simulink model "IEEE123bus_v2019b_Phasor_PI"  (R2019b)
settings: Solver=ode4  StartTime=0.0  StopTime=100  FixedStep=Ts  MaxStep=1e-4  RelTol=1e-3
InitFcn:
  | a=1; % Loading Factor
  | Ts=0.1;% For Delay Blocks in Voltage Regulator Controls
  | % phase to sequence conversion of RXB matrices
  | c=1*exp(sqrt(-1)*(120*pi/180));
  | T=[1 1 1;1 c*c c;1 c c*c];
  | Tinv=1/3*[1 1 1;1 c c*c;1 c*c c];
  | 
  | % Simulation data for the IEEE 123 Node Test Feeder model
  | mi2km = 1.60934;%  miles to km conversion
  | ft2km = 0.0003048; % feet to km conversion
  | ms2F = 1*1e-6/(2*pi*60);% microsiemens to Farads conversion
  | 
  | %% Configuration 1
  | % Series Resitance and Reactance - ohm/mile
  | R_1 = [0.4576 0.1560 0.1535;0.1560 0.4666 0.1580;0.1535 0.1580 0.4615];
  | X_1 = [1.0780 0.5017 0.3849;0.5017 1.0482 0.4236;0.3849 0.4236 1.0651];
  | % charging susceptance - microsiemens/mile
  | B_1 = [5.6765 -1.8319 -0.6982;-1.8319 5.9809 -1.1645;-0.6982 -1.1645 5.3971];
  | 
  | R_1 = R_1/mi2km;
  | Rseq=Tinv*R_1*T;
  | R1_1=Rseq(2,2);R0_1=Rseq(1,1);
  | 
  | L_1 = (X_1/(2*pi*60))/mi2km;
  | Lseq=Tinv*L_1*T;
  | L1_1=Lseq(2,2);L0_1=Lseq(1,1);
  | 
  | C_1 =(B_1*ms2F)/mi2km;
  | Cseq=Tinv*C_1*T;
  | C1_1=Cseq(2,2);C0_1=Cseq(1,1);
  | %% Configuration 2 - series reactance - ohm/mile
  | R_2 = [0.4666 0.1580 0.1560;0.1580 0.4615 0.1535;0.1560 0.1535 0.4576];
  | X_2 = [1.0482 0.4236 0.5017;0.4236 1.0651 0.3849;0.5017 0.3849 1.0780];
  | % charging susceptance - microsiemens/mile
  | B_2 = [5.9809 -1.1645 -1.8319;-1.1645 5.3971 -0.6982;-1.8319 -0.6982 5.6765];
  | 
  | R_2 = R_2/mi2km;
  | Rseq=Tinv*R_2*T;
  | R1_2=Rseq(2,2);R0_2=Rseq(1,1);
  | 
  | L_2 = (X_2/(2*pi*60))/mi2km;
  | Lseq=Tinv*L_2*T;
  | L1_2=Lseq(2,2);L0_2=Lseq(1,1);
  | 
  | C_2 =(B_2*ms2F)/mi2km;
  | Cseq=Tinv*C_2*T;
  | C1_2=Cseq(2,2);C0_2=Cseq(1,1);
  | %% Configuration 3 - series reactance - ohm/mile
  | R_3 = [0.4615 0.1535 0.1580;0.1535 0.4576 0.1560;0.1580 0.1560 0.4666];
  | X_3 = [1.0651 0.3849 0.4236;0.3849 1.0780 0.5017;0.4236 0.5017 1.0482];
  | % charging susceptance - microsiemens/mile
  | B_3 = [5.3971 -0.6982 -1.1645;-0.6982 5.6765 -1.8319; -1.1645 -1.8319 5.9809];
  | 
  | R_3 = R_3/mi2km;
  | Rseq=Tinv*R_3*T;
  | R1_3=Rseq(2,2);R0_3=Rseq(1,1);
  | 
  | L_3 = (X_3/(2*pi*60))/mi2km;
  | Lseq=Tinv*L_3*T;
  | L1_3=Lseq(2,2);L0_3=Lseq(1,1);
  | ... (+157 lines)
undefined symbols (not defined in the file or in its folder): D1, Delta, find_system, j
libraries: powerlib x771, powerlib_meascontrol x31
(part 4 of 7)

== system IEEE123bus_v2019b_Phasor_PI/Regulator 3 ==
  Mux : Mux  Inputs=2
  Single Phase SVR_A : Subsystem  LoadFcn=find_system(gcs,'FollowLinks', 'on', 'LookUnderMasks', 'all');  mask(Single-Phase OLTC){pNom=5e6/3, fNom=60, vNom=4160/sqrt(3), ctRatio=50, ptRatio=20, DeltaU=0.00625, TapMinMax=[-16 16], InitialTap=0, TapSelectionTime=8, RegulatorOn=on, Regulator=[120/120  1/120  12], Comp=[0.4 0.4]}
      mask prompts: pNom "Nominal Power (VA)"; fNom "Nominal Frequency (Hz)"; vNom "Nominal Voltage (Vrms)"; ctRatio "Primary CT Rating (A)"; ptRatio "PT Ratio"; DeltaU "Voltage Step Per Tap (pu)"; TapMinMax "Minimum and Maximum Tap Positions"; InitialTap "Initial Tap Position"; TapSelectionTime "Tap Selection Time (s)"; RegulatorOn "Voltage Regulator"; Regulator "Voltage Regulator [ Vref(pu) DeadBand(pu)  Delay(s)]"; Comp "Compensator Settings [R (V) X(V)]"
      mask help:
      | Models a single-phase On Load Tap Changer (OLTC). The single-phase primary of multi-tap winding is modeled with a Variable-Ratio Transformer block.
      |
      | The transformer voltage ratio U2/U1 (in pu) is given by:
      |                 U2/U1= 1/ (1+TapPosition*DeltaU)
      | Tap position 0 corresponds to nominal voltage ratio.
      |
      | When Voltage regulator is 'on',  voltage regulator asks for a tap change if:
      |                  abs(Vm-Vref)>DeadBand/2  during a time  t > Delay.
      |
      | where 'Vm' is voltage measured at regulating point and Vref is reference voltage.
      | With line drop compensation, Vm=Vsec-Isec(R+jX)
      mask init:
      | RegulatorVref=Regulator(1);
      | RegulatorDeadBand=Regulator(2);
      | RegulatorDelay=Regulator(3);
      | Rc=Comp(1);
      | Xc=Comp(2);
      mask TypeOptions RegulatorOn: off | on
      mask Callback RegulatorOn:
      | tempMaskVis=get_param(gcb,'MaskVisibilities');
      | if strcmp(get_param(gcb,'RegulatorOn'),'on')
      | 	tempMaskVis{11}='on';
      | 	set_param(gcb,'MaskVisibilities',tempMaskVis);
      | else
      | 	tempMaskVis{11}='off';
      | 	set_param(gcb,'MaskVisibilities',tempMaskVis);
      | end
      | if strcmp(get_param(gcb,'RegulatorOn'),'on')
      | 	tempMaskVis{12}='on';
      | 	set_param(gcb,'MaskVisibilities',tempMaskVis);
      | else
      | 	tempMaskVis{12}='off';
      | 	set_param(gcb,'MaskVisibilities',tempMaskVis);
      | end
      mask DialogControl Container8 Prompt: Setup
      mask DialogControl Container13 Prompt: Regulator Parameters
  Single Phase SVR_C : Subsystem  LoadFcn=find_system(gcs,'FollowLinks', 'on', 'LookUnderMasks', 'all');  mask(Single-Phase OLTC){pNom=5e6/3, fNom=60, vNom=4160/sqrt(3), ctRatio=50, ptRatio=20, DeltaU=0.00625, TapMinMax=[-16 16], InitialTap=-1, TapSelectionTime=8, RegulatorOn=on, Regulator=[120/120  1/120  12], Comp=[0.4 0.4]}
      mask prompts: pNom "Nominal Power (VA)"; fNom "Nominal Frequency (Hz)"; vNom "Nominal Voltage (Vrms)"; ctRatio "Primary CT Rating (A)"; ptRatio "PT Ratio"; DeltaU "Voltage Step Per Tap (pu)"; TapMinMax "Minimum and Maximum Tap Positions"; InitialTap "Initial Tap Position"; TapSelectionTime "Tap Selection Time (s)"; RegulatorOn "Voltage Regulator"; Regulator "Voltage Regulator [ Vref(pu) DeadBand(pu)  Delay(s)]"; Comp "Compensator Settings [R (V) X(V)]"
      mask help:
      | Models a single-phase On Load Tap Changer (OLTC). The single-phase primary of multi-tap winding is modeled with a Variable-Ratio Transformer block.
      |
      | The transformer voltage ratio U2/U1 (in pu) is given by:
      |                 U2/U1= 1/ (1+TapPosition*DeltaU)
      | Tap position 0 corresponds to nominal voltage ratio.
      |
      | When Voltage regulator is 'on',  voltage regulator asks for a tap change if:
      |                  abs(Vm-Vref)>DeadBand/2  during a time  t > Delay.
      |
      | where 'Vm' is voltage measured at regulating point and Vref is reference voltage.
      | With line drop compensation, Vm=Vsec-Isec(R+jX)
      mask init:
      | RegulatorVref=Regulator(1);
      | RegulatorDeadBand=Regulator(2);
      | RegulatorDelay=Regulator(3);
      | Rc=Comp(1);
      | Xc=Comp(2);
      mask TypeOptions RegulatorOn: off | on
      mask Callback RegulatorOn:
      | tempMaskVis=get_param(gcb,'MaskVisibilities');
      | if strcmp(get_param(gcb,'RegulatorOn'),'on')
      | 	tempMaskVis{11}='on';
      | 	set_param(gcb,'MaskVisibilities',tempMaskVis);
      | else
      | 	tempMaskVis{11}='off';
      | 	set_param(gcb,'MaskVisibilities',tempMaskVis);
      | end
      | if strcmp(get_param(gcb,'RegulatorOn'),'on')
      | 	tempMaskVis{12}='on';
      | 	set_param(gcb,'MaskVisibilities',tempMaskVis);
      | else
      | 	tempMaskVis{12}='off';
      | 	set_param(gcb,'MaskVisibilities',tempMaskVis);
      | end
      mask DialogControl Container8 Prompt: Setup
      mask DialogControl Container13 Prompt: Regulator Parameters
  A : PMIOPort  Side=Left
  a : PMIOPort  Port=2  Side=Right
  C : PMIOPort  Port=3  Side=Left
  c : PMIOPort  Port=4  Side=Right
  Taps : Outport
  wires:
  Single Phase SVR_A/1(Tap) -> Mux/1
  Single Phase SVR_C/1(Tap) -> Mux/2
  Mux/1 -> Taps/1
  connections:
  Single Phase SVR_A/LConn1 -- A/RConn1
  Single Phase SVR_C/LConn1 -- C/RConn1
  Single Phase SVR_A/RConn1 -- a/RConn1
  Single Phase SVR_C/RConn1 -- c/RConn1

== system IEEE123bus_v2019b_Phasor_PI/Regulator 4 ==
  Mux : Mux  Inputs=3
  Single Phase SVR_A : Subsystem  LoadFcn=find_system(gcs,'FollowLinks', 'on', 'LookUnderMasks', 'all');  mask(Single-Phase OLTC){pNom=5e6/3, fNom=60, vNom=4160/sqrt(3), ctRatio=300, ptRatio=20, DeltaU=0.00625, TapMinMax=[-16 16], InitialTap=8, TapSelectionTime=8, RegulatorOn=on, Regulator=[124/120  2/120  12], Comp=[0.6 1.3]}
      mask prompts: pNom "Nominal Power (VA)"; fNom "Nominal Frequency (Hz)"; vNom "Nominal Voltage (Vrms)"; ctRatio "Primary CT Rating (A)"; ptRatio "PT Ratio"; DeltaU "Voltage Step Per Tap (pu)"; TapMinMax "Minimum and Maximum Tap Positions"; InitialTap "Initial Tap Position"; TapSelectionTime "Tap Selection Time (s)"; RegulatorOn "Voltage Regulator"; Regulator "Voltage Regulator [ Vref(pu) DeadBand(pu)  Delay(s)]"; Comp "Compensator Settings [R (V) X(V)]"
      mask help:
      | Models a single-phase On Load Tap Changer (OLTC). The single-phase primary of multi-tap winding is modeled with a Variable-Ratio Transformer block.
      |
      | The transformer voltage ratio U2/U1 (in pu) is given by:
      |                 U2/U1= 1/ (1+TapPosition*DeltaU)
      | Tap position 0 corresponds to nominal voltage ratio.
      |
      | When Voltage regulator is 'on',  voltage regulator asks for a tap change if:
      |                  abs(Vm-Vref)>DeadBand/2  during a time  t > Delay.
      |
      | where 'Vm' is voltage measured at regulating point and Vref is reference voltage.
      | With line drop compensation, Vm=Vsec-Isec(R+jX)
      mask init:
      | RegulatorVref=Regulator(1);
      | RegulatorDeadBand=Regulator(2);
      | RegulatorDelay=Regulator(3);
      | Rc=Comp(1);
      | Xc=Comp(2);
      mask TypeOptions RegulatorOn: off | on
      mask Callback RegulatorOn:
      | tempMaskVis=get_param(gcb,'MaskVisibilities');
      | if strcmp(get_param(gcb,'RegulatorOn'),'on')
      | 	tempMaskVis{11}='on';
      | 	set_param(gcb,'MaskVisibilities',tempMaskVis);
      | else
      | 	tempMaskVis{11}='off';
      | 	set_param(gcb,'MaskVisibilities',tempMaskVis);
      | end
      | if strcmp(get_param(gcb,'RegulatorOn'),'on')
      | 	tempMaskVis{12}='on';
      | 	set_param(gcb,'MaskVisibilities',tempMaskVis);
      | else
      | 	tempMaskVis{12}='off';
      | 	set_param(gcb,'MaskVisibilities',tempMaskVis);
      | end
      mask DialogControl Container8 Prompt: Setup
      mask DialogControl Container13 Prompt: Regulator Parameters
  Single Phase SVR_B : Subsystem  LoadFcn=find_system(gcs,'FollowLinks', 'on', 'LookUnderMasks', 'all');  mask(Single-Phase OLTC){pNom=5e6/3, fNom=60, vNom=4160/sqrt(3), ctRatio=300, ptRatio=20, DeltaU=0.00625, TapMinMax=[-16 16], InitialTap=1, TapSelectionTime=8, RegulatorOn=on, Regulator=[124/120  2/120  12], Comp=[0.6 1.3]}
      mask prompts: pNom "Nominal Power (VA)"; fNom "Nominal Frequency (Hz)"; vNom "Nominal Voltage (Vrms)"; ctRatio "Primary CT Rating (A)"; ptRatio "PT Ratio"; DeltaU "Voltage Step Per Tap (pu)"; TapMinMax "Minimum and Maximum Tap Positions"; InitialTap "Initial Tap Position"; TapSelectionTime "Tap Selection Time (s)"; RegulatorOn "Voltage Regulator"; Regulator "Voltage Regulator [ Vref(pu) DeadBand(pu)  Delay(s)]"; Comp "Compensator Settings [R (V) X(V)]"
      mask help:
      | Models a single-phase On Load Tap Changer (OLTC). The single-phase primary of multi-tap winding is modeled with a Variable-Ratio Transformer block.
      |
      | The transformer voltage ratio U2/U1 (in pu) is given by:
      |                 U2/U1= 1/ (1+TapPosition*DeltaU)
      | Tap position 0 corresponds to nominal voltage ratio.
      |
      | When Voltage regulator is 'on',  voltage regulator asks for a tap change if:
      |                  abs(Vm-Vref)>DeadBand/2  during a time  t > Delay.
      |
      | where 'Vm' is voltage measured at regulating point and Vref is reference voltage.
      | With line drop compensation, Vm=Vsec-Isec(R+jX)
      mask init:
      | RegulatorVref=Regulator(1);
      | RegulatorDeadBand=Regulator(2);
      | RegulatorDelay=Regulator(3);
      | Rc=Comp(1);
      | Xc=Comp(2);
      mask TypeOptions RegulatorOn: off | on
      mask Callback RegulatorOn:
      | tempMaskVis=get_param(gcb,'MaskVisibilities');
      | if strcmp(get_param(gcb,'RegulatorOn'),'on')
      | 	tempMaskVis{11}='on';
      | 	set_param(gcb,'MaskVisibilities',tempMaskVis);
      | else
      | 	tempMaskVis{11}='off';
      | 	set_param(gcb,'MaskVisibilities',tempMaskVis);
      | end
      | if strcmp(get_param(gcb,'RegulatorOn'),'on')
      | 	tempMaskVis{12}='on';
      | 	set_param(gcb,'MaskVisibilities',tempMaskVis);
      | else
      | 	tempMaskVis{12}='off';
      | 	set_param(gcb,'MaskVisibilities',tempMaskVis);
      | end
      mask DialogControl Container8 Prompt: Setup
      mask DialogControl Container13 Prompt: Regulator Parameters
  Single Phase SVR_C : Subsystem  LoadFcn=find_system(gcs,'FollowLinks', 'on', 'LookUnderMasks', 'all');  mask(Single-Phase OLTC){pNom=5e6/3, fNom=60, vNom=4160/sqrt(3), ctRatio=300, ptRatio=20, DeltaU=0.00625, TapMinMax=[-16 16], InitialTap=5, TapSelectionTime=8, RegulatorOn=on, Regulator=[124/120  2/120  12], Comp=[0.6 1.3]}
      mask prompts: pNom "Nominal Power (VA)"; fNom "Nominal Frequency (Hz)"; vNom "Nominal Voltage (Vrms)"; ctRatio "Primary CT Rating (A)"; ptRatio "PT Ratio"; DeltaU "Voltage Step Per Tap (pu)"; TapMinMax "Minimum and Maximum Tap Positions"; InitialTap "Initial Tap Position"; TapSelectionTime "Tap Selection Time (s)"; RegulatorOn "Voltage Regulator"; Regulator "Voltage Regulator [ Vref(pu) DeadBand(pu)  Delay(s)]"; Comp "Compensator Settings [R (V) X(V)]"
      mask help:
      | Models a single-phase On Load Tap Changer (OLTC). The single-phase primary of multi-tap winding is modeled with a Variable-Ratio Transformer block.
      |
      | The transformer voltage ratio U2/U1 (in pu) is given by:
      |                 U2/U1= 1/ (1+TapPosition*DeltaU)
      | Tap position 0 corresponds to nominal voltage ratio.
      |
      | When Voltage regulator is 'on',  voltage regulator asks for a tap change if:
      |                  abs(Vm-Vref)>DeadBand/2  during a time  t > Delay.
      |
      | where 'Vm' is voltage measured at regulating point and Vref is reference voltage.
      | With line drop compensation, Vm=Vsec-Isec(R+jX)
      mask init:
      | RegulatorVref=Regulator(1);
      | RegulatorDeadBand=Regulator(2);
      | RegulatorDelay=Regulator(3);
      | Rc=Comp(1);
      | Xc=Comp(2);
      mask TypeOptions RegulatorOn: off | on
      mask Callback RegulatorOn:
      | tempMaskVis=get_param(gcb,'MaskVisibilities');
      | if strcmp(get_param(gcb,'RegulatorOn'),'on')
      | 	tempMaskVis{11}='on';
      | 	set_param(gcb,'MaskVisibilities',tempMaskVis);
      | else
      | 	tempMaskVis{11}='off';
      | 	set_param(gcb,'MaskVisibilities',tempMaskVis);
      | end
      | if strcmp(get_param(gcb,'RegulatorOn'),'on')
      | 	tempMaskVis{12}='on';
      | 	set_param(gcb,'MaskVisibilities',tempMaskVis);
      | else
      | 	tempMaskVis{12}='off';
      | 	set_param(gcb,'MaskVisibilities',tempMaskVis);
      | end
      mask DialogControl Container8 Prompt: Setup
      mask DialogControl Container13 Prompt: Regulator Parameters
  A : PMIOPort  Side=Left
  a : PMIOPort  Port=2  Side=Right
  B : PMIOPort  Port=3  Side=Left
  b : PMIOPort  Port=4  Side=Right
  C : PMIOPort  Port=5  Side=Left
  c : PMIOPort  Port=6  Side=Right
  Tap : Outport
  wires:
  Mux/1 -> Tap/1
  Single Phase SVR_C/1(Tap) -> Mux/3
  Single Phase SVR_B/1(Tap) -> Mux/2
  Single Phase SVR_A/1(Tap) -> Mux/1
  connections:
  Single Phase SVR_C/RConn1 -- c/RConn1
  Single Phase SVR_C/LConn1 -- C/RConn1
  Single Phase SVR_B/RConn1 -- b/RConn1
  Single Phase SVR_B/LConn1 -- B/RConn1
  Single Phase SVR_A/LConn1 -- A/RConn1
  Single Phase SVR_A/RConn1 -- a/RConn1

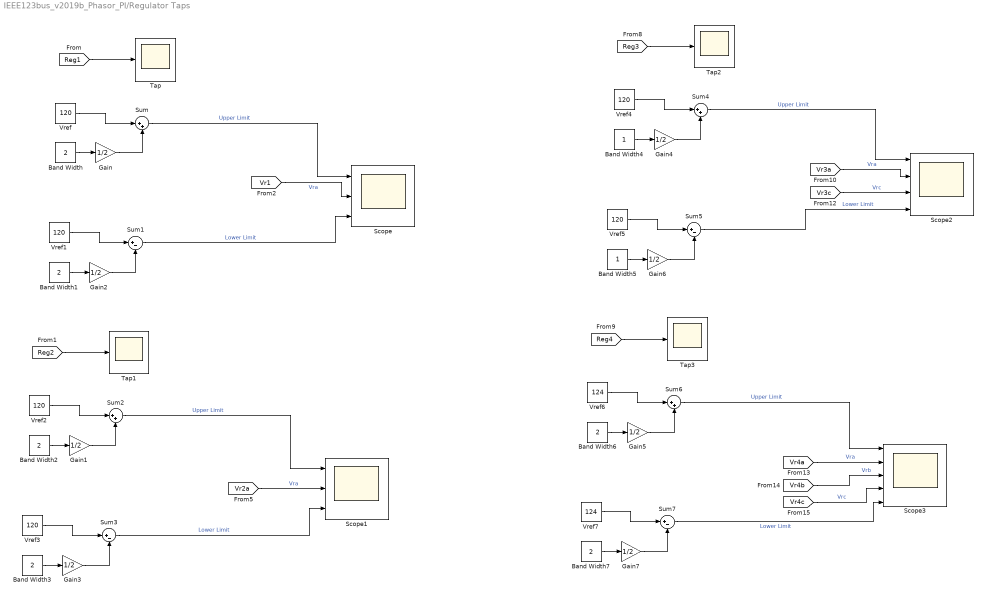
== system IEEE123bus_v2019b_Phasor_PI/Regulator Taps ==
  Band Width{,1..3,6..7} (6 alike) : Constant  Value=2
  Band Width4 : Constant
  Band Width5 : Constant
  Gain{,1..7} (8 alike) : Gain  Gain=1/2
  Scope : Scope  NumInputPorts=3
  Scope1 : Scope  NumInputPorts=3
  Scope2 : Scope  NumInputPorts=4
  Scope3 : Scope  NumInputPorts=5
  Sum{,2,4,6} (4 alike) : Sum  Inputs=|++
  Sum{1,3,5,7} (4 alike) : Sum  Inputs=|+-
  Tap{,1..3} (4 alike) : Scope
  Vref{,1..5} (6 alike) : Constant  Value=120
  Vref6 : Constant  Value=124
  Vref7 : Constant  Value=124
  wires:
  Vref/1 -> Sum/1
  Gain2/1 -> Sum1/2
  Band Width/1 -> Gain/1
  Gain/1 -> Sum/2
  [Reg1] -> Tap/1
  Band Width1/1 -> Gain2/1
  Sum/1 -> Scope/1  "Upper Limit"
  Vref1/1 -> Sum1/1
  Sum1/1 -> Scope/3  "Lower Limit"
  [Vr1] -> Scope/2  "Vra"
  [Vr2a] -> Scope1/2  "Vra"
  Sum3/1 -> Scope1/3  "Lower Limit"
  Vref3/1 -> Sum3/1
  Sum2/1 -> Scope1/1  "Upper Limit"
  Band Width3/1 -> Gain3/1
  [Reg2] -> Tap1/1
  Gain1/1 -> Sum2/2
  Band Width2/1 -> Gain1/1
  Gain3/1 -> Sum3/2
  Vref2/1 -> Sum2/1
  Vref6/1 -> Sum6/1
  Gain7/1 -> Sum7/2
  Band Width6/1 -> Gain5/1
  Gain5/1 -> Sum6/2
  [Reg4] -> Tap3/1
  [Vr4c] -> Scope3/4  "Vrc"
  Band Width7/1 -> Gain7/1
  Sum6/1 -> Scope3/1  "Upper Limit"
  Vref7/1 -> Sum7/1
  Sum7/1 -> Scope3/5  "Lower Limit"
  [Vr4b] -> Scope3/3  "Vrb"
  [Vr4a] -> Scope3/2  "Vra"
  [Vr3a] -> Scope2/2  "Vra"
  Sum5/1 -> Scope2/4  "Lower Limit"
  Vref5/1 -> Sum5/1
  Sum4/1 -> Scope2/1  "Upper Limit"
  Band Width5/1 -> Gain6/1
  [Vr3c] -> Scope2/3  "Vrc"
  [Reg3] -> Tap2/1
  Gain4/1 -> Sum4/2
  Band Width4/1 -> Gain4/1
  Gain6/1 -> Sum5/2
  Vref4/1 -> Sum4/1

== system IEEE123bus_v2019b_Phasor_PI/Substation Power ==
  note: TOTAL
  note: From Benchmark Document
      |
      | SYSTEM PHASE PHASE PHASE TOTAL
      | INPUT -------(A)-------|-------(B)-------|-------(C)-------|------------------
      | kW : 1463.861 | 963.484 | 1193.153 | 3620.498
      | kVAr : 582.101 | 343.687 | 398.976 | 1324.765
  note: PHASE A
  note: PHASE B
  note: PHASE C
  Demux : Demux  Outputs=3
  Demux1 : Demux  Outputs=3
  Display{,1..7} (8 alike) : Display
  Gain{,1..7} (8 alike) : Gain  Gain=1e-3
  "Power (3ph, Phasor)" : powerlib_meascontrol/Measurements/Power (3ph, Phasor)
      settings: SourceProductName=Simscape Electrical  SourceProductBaseCode=PS
  Power (Phasor) : powerlib_meascontrol/Measurements/Power (Phasor)
      settings: SourceProductName=Simscape Electrical  SourceProductBaseCode=PS
  Power (Phasor)1 : powerlib_meascontrol/Measurements/Power (Phasor)
      settings: SourceProductName=Simscape Electrical  SourceProductBaseCode=PS
  Power (Phasor)2 : powerlib_meascontrol/Measurements/Power (Phasor)
      settings: SourceProductName=Simscape Electrical  SourceProductBaseCode=PS
  wires:
  [I150] -> "Power (3ph, Phasor)"/2
  [V150] -> "Power (3ph, Phasor)"/1
  "Power (3ph, Phasor)"/1 -> Gain/1
  "Power (3ph, Phasor)"/2 -> Gain1/1
  [V150] -> Demux/1
  [I150] -> Demux1/1
  Demux/1 -> Power (Phasor)/1
  Demux1/1 -> Power (Phasor)/2
  Demux/2 -> Power (Phasor)1/1
  Demux1/2 -> Power (Phasor)1/2
  Demux/3 -> Power (Phasor)2/1
  Demux1/3 -> Power (Phasor)2/2
  Power (Phasor)/1 -> Gain2/1
  Power (Phasor)/2 -> Gain3/1
  Power (Phasor)1/1 -> Gain4/1
  Power (Phasor)1/2 -> Gain5/1
  Power (Phasor)2/1 -> Gain6/1
  Power (Phasor)2/2 -> Gain7/1
  Gain/1 -> Display/1
  Gain1/1 -> Display1/1
  Gain2/1 -> Display2/1
  Gain3/1 -> Display3/1
  Gain4/1 -> Display4/1
  Gain5/1 -> Display5/1
  Gain6/1 -> Display6/1
  Gain7/1 -> Display7/1

== system IEEE123bus_v2019b_Phasor_PI/Regulator 1/Single Phase SVR_A ==
  Line Drop Compensator : Subsystem
  Transformer with Taps : Subsystem
  Voltage Regulator Control : Subsystem
  S : PMIOPort  Tag=PMCPort  Side=Left
  L : PMIOPort  Tag=PMCPort  Port=2  Side=Right
  Tap : Outport  VectorParamsAs1DForOutWhenUnconnected=off
  tag scope: Vr2a=global
  wires:
  Line Drop Compensator/1(Vm) -> Voltage Regulator Control/1(Vm), [Vr2a]
  Voltage Regulator Control/1(Tap) -> Transformer with Taps/1(tap), Tap/1
  Transformer with Taps/1(Isec) -> Line Drop Compensator/1(Isec)
  Transformer with Taps/2(Vsec) -> Line Drop Compensator/2(Vsec)
  connections:
  Transformer with Taps/RConn1 -- L/RConn1
  Transformer with Taps/LConn1 -- S/RConn1

== system IEEE123bus_v2019b_Phasor_PI/Regulator 1 Three Phase Ganged SVR/Ganged Line Drop Compensator ==
  note: Vm=Vsec-Isec(Rc+jXc)
  Isec : Inport
  Vsec : Inport  Port=2
  Abs1 : Abs
  Gain4 : Gain  Gain=1/sqrt(2)
  Gain5 : Gain  Gain=Rc+j*Xc
  Gain6 : Gain  Gain=1/sqrt(2)
  Sum1 : Sum  Inputs=|+-
  Vm : Outport
  wires:
  Abs1/1 -> Vm/1
  Gain5/1 -> Sum1/2
  Isec/1 -> Gain4/1
  Gain4/1 -> Gain5/1
  Gain6/1 -> Sum1/1
  Sum1/1 -> Abs1/1
  Vsec/1 -> Gain6/1

== system IEEE123bus_v2019b_Phasor_PI/Regulator 1 Three Phase Ganged SVR/Single Phase SVR_A ==
  Vm : Inport
  Transformer with Taps : Subsystem
  Voltage Regulator Control : Subsystem
  S : PMIOPort  Tag=PMCPort  Side=Left
  L : PMIOPort  Tag=PMCPort  Port=2  Side=Right
  Tap : Outport  VectorParamsAs1DForOutWhenUnconnected=off
  Isec : Outport  Port=2  VectorParamsAs1DForOutWhenUnconnected=off
  Vsec : Outport  Port=3  VectorParamsAs1DForOutWhenUnconnected=off
  wires:
  Transformer with Taps/2(Vsec) -> Vsec/1
  Transformer with Taps/1(Isec) -> Isec/1
  Voltage Regulator Control/1(Tap) -> Transformer with Taps/1(tap), Tap/1
  Vm/1 -> Voltage Regulator Control/1(Vm)
  connections:
  Transformer with Taps/LConn1 -- S/RConn1
  Transformer with Taps/RConn1 -- L/RConn1

== system IEEE123bus_v2019b_Phasor_PI/Regulator 1 Three Phase Ganged SVR/Single Phase SVR_B ==
  Vm : Inport
  Transformer with Taps : Subsystem
  Voltage Regulator Control : Subsystem
  S : PMIOPort  Tag=PMCPort  Side=Left
  L : PMIOPort  Tag=PMCPort  Port=2  Side=Right
  Tap : Outport  VectorParamsAs1DForOutWhenUnconnected=off
  Isec : Outport  Port=2  VectorParamsAs1DForOutWhenUnconnected=off
  Vsec : Outport  Port=3  VectorParamsAs1DForOutWhenUnconnected=off
  wires:
  Vm/1 -> Voltage Regulator Control/1(Vm)
  Voltage Regulator Control/1(Tap) -> Transformer with Taps/1(tap), Tap/1
  Transformer with Taps/1(Isec) -> Isec/1
  Transformer with Taps/2(Vsec) -> Vsec/1
  connections:
  Transformer with Taps/RConn1 -- L/RConn1
  Transformer with Taps/LConn1 -- S/RConn1

== system IEEE123bus_v2019b_Phasor_PI/Regulator 1 Three Phase Ganged SVR/Single Phase SVR_C ==
  Vm : Inport
  Transformer with Taps : Subsystem
  Voltage Regulator Control : Subsystem
  S : PMIOPort  Tag=PMCPort  Side=Left
  L : PMIOPort  Tag=PMCPort  Port=2  Side=Right
  Tap : Outport  VectorParamsAs1DForOutWhenUnconnected=off
  Isec : Outport  Port=2  VectorParamsAs1DForOutWhenUnconnected=off
  Vsec : Outport  Port=3  VectorParamsAs1DForOutWhenUnconnected=off
  wires:
  Transformer with Taps/2(Vsec) -> Vsec/1
  Transformer with Taps/1(Isec) -> Isec/1
  Voltage Regulator Control/1(Tap) -> Transformer with Taps/1(tap), Tap/1
  Vm/1 -> Voltage Regulator Control/1(Vm)
  connections:
  Transformer with Taps/LConn1 -- S/RConn1
  Transformer with Taps/RConn1 -- L/RConn1

== system IEEE123bus_v2019b_Phasor_PI/Regulator 3/Single Phase SVR_A ==
  Line Drop Compensator : Subsystem
  Transformer with Taps : Subsystem
  Voltage Regulator Control : Subsystem
  S : PMIOPort  Tag=PMCPort  Side=Left
  L : PMIOPort  Tag=PMCPort  Port=2  Side=Right
  Tap : Outport  VectorParamsAs1DForOutWhenUnconnected=off
  tag scope: Vr3a=global
  wires:
  Line Drop Compensator/1(Vm) -> Voltage Regulator Control/1(Vm), [Vr3a]
  Voltage Regulator Control/1(Tap) -> Transformer with Taps/1(tap), Tap/1
  Transformer with Taps/1(Isec) -> Line Drop Compensator/1(Isec)
  Transformer with Taps/2(Vsec) -> Line Drop Compensator/2(Vsec)
  connections:
  Transformer with Taps/RConn1 -- L/RConn1
  Transformer with Taps/LConn1 -- S/RConn1

== system IEEE123bus_v2019b_Phasor_PI/Regulator 3/Single Phase SVR_C ==
  Line Drop Compensator : Subsystem
  Transformer with Taps : Subsystem
  Voltage Regulator Control : Subsystem
  S : PMIOPort  Tag=PMCPort  Side=Left
  L : PMIOPort  Tag=PMCPort  Port=2  Side=Right
  Tap : Outport  VectorParamsAs1DForOutWhenUnconnected=off
  tag scope: Vr3c=global
  wires:
  Transformer with Taps/2(Vsec) -> Line Drop Compensator/2(Vsec)
  Transformer with Taps/1(Isec) -> Line Drop Compensator/1(Isec)
  Voltage Regulator Control/1(Tap) -> Transformer with Taps/1(tap), Tap/1
  Line Drop Compensator/1(Vm) -> Voltage Regulator Control/1(Vm), [Vr3c]
  connections:
  Transformer with Taps/LConn1 -- S/RConn1
  Transformer with Taps/RConn1 -- L/RConn1

== system IEEE123bus_v2019b_Phasor_PI/Regulator 4/Single Phase SVR_A ==
  Line Drop Compensator : Subsystem
  Transformer with Taps : Subsystem
  Voltage Regulator Control : Subsystem
  S : PMIOPort  Tag=PMCPort  Side=Left
  L : PMIOPort  Tag=PMCPort  Port=2  Side=Right
  Tap : Outport  VectorParamsAs1DForOutWhenUnconnected=off
  tag scope: Vr4a=global
  wires:
  Line Drop Compensator/1(Vm) -> Voltage Regulator Control/1(Vm), [Vr4a]
  Voltage Regulator Control/1(Tap) -> Tap/1, Transformer with Taps/1(tap)
  Transformer with Taps/1(Isec) -> Line Drop Compensator/1(Isec)
  Transformer with Taps/2(Vsec) -> Line Drop Compensator/2(Vsec)
  connections:
  Transformer with Taps/RConn1 -- L/RConn1
  Transformer with Taps/LConn1 -- S/RConn1

== system IEEE123bus_v2019b_Phasor_PI/Regulator 4/Single Phase SVR_B ==
  Line Drop Compensator : Subsystem
  Transformer with Taps : Subsystem
  Voltage Regulator Control : Subsystem
  S : PMIOPort  Tag=PMCPort  Side=Left
  L : PMIOPort  Tag=PMCPort  Port=2  Side=Right
  Tap : Outport  VectorParamsAs1DForOutWhenUnconnected=off
  tag scope: Vr4b=global
  wires:
  Transformer with Taps/2(Vsec) -> Line Drop Compensator/2(Vsec)
  Transformer with Taps/1(Isec) -> Line Drop Compensator/1(Isec)
  Voltage Regulator Control/1(Tap) -> Transformer with Taps/1(tap), Tap/1
  Line Drop Compensator/1(Vm) -> Voltage Regulator Control/1(Vm), [Vr4b]
  connections:
  Transformer with Taps/LConn1 -- S/RConn1
  Transformer with Taps/RConn1 -- L/RConn1

== system IEEE123bus_v2019b_Phasor_PI/Regulator 4/Single Phase SVR_C ==
  Line Drop Compensator : Subsystem
  Transformer with Taps : Subsystem
  Voltage Regulator Control : Subsystem
  S : PMIOPort  Tag=PMCPort  Side=Left
  L : PMIOPort  Tag=PMCPort  Port=2  Side=Right
  Tap : Outport  VectorParamsAs1DForOutWhenUnconnected=off
  tag scope: Vr4c=global
  wires:
  Line Drop Compensator/1(Vm) -> Voltage Regulator Control/1(Vm), [Vr4c]
  Voltage Regulator Control/1(Tap) -> Transformer with Taps/1(tap), Tap/1
  Transformer with Taps/1(Isec) -> Line Drop Compensator/1(Isec)
  Transformer with Taps/2(Vsec) -> Line Drop Compensator/2(Vsec)
  connections:
  Transformer with Taps/RConn1 -- L/RConn1
  Transformer with Taps/LConn1 -- S/RConn1

== system IEEE123bus_v2019b_Phasor_PI/Regulator 1/Single Phase SVR_A/Line Drop Compensator ==
  note: Vm=Vsec-Isec(Rc+jXc)
  Isec : Inport
  Vsec : Inport  Port=2
  Abs1 : Abs
  Gain4 : Gain  Gain=1/sqrt(2)
  Gain5 : Gain  Gain=Rc+j*Xc
  Gain6 : Gain  Gain=1/sqrt(2)
  Sum1 : Sum  Inputs=|+-
  Vm : Outport
  wires:
  Gain5/1 -> Sum1/2
  Gain6/1 -> Sum1/1
  Gain4/1 -> Gain5/1
  Vsec/1 -> Gain6/1
  Isec/1 -> Gain4/1
  Sum1/1 -> Abs1/1
  Abs1/1 -> Vm/1

== system IEEE123bus_v2019b_Phasor_PI/Regulator 1/Single Phase SVR_A/Transformer with Taps ==
  note: Isec on CT Ratio base
  note: Vsec on Pt Ratio base
  tap : Inport
  "    " : Gain  Gain=(1/ptRatio)
  " 1" : Gain  Gain=(1/ctRatio)
  CT : powerlib/Measurements/Current Measurement  PhasorSimulation=on  OutputType=Complex  PSBequivalent=0
      settings: SourceProductName=Simscape Electrical
  Ground1 : powerlib/Elements/Ground  LConnTagsString=a
      settings: SourceProductName=Simscape Electrical
  Ground2 : powerlib/Elements/Ground  LConnTagsString=a
      settings: SourceProductName=Simscape Electrical
  Ground3 : powerlib/Elements/Ground  LConnTagsString=a
      settings: SourceProductName=Simscape Electrical
  Memory : Memory
  Memory1 : Memory
  PT : powerlib/Measurements/Voltage Measurement  PhasorSimulation=on  OutputType=Complex  PSBequivalent=0
      settings: SourceProductName=Simscape Electrical
  Tap Changing Transformer : Subsystem  mask(Tap Changing Transformer){}
      mask help: Implements a Tap changing two-winding ideal transformer with taps at secondary.
      mask Display:
      | A=[-85 -45 -44 -34 -26 -21 -20 -22 -28 -37 -47 -57 -63 -63 -54 -44 -34 -26 -21 -20 -22 -28 -37 -47 -57 -63 -63 -54 -44 -34 -26 -21 -20 -22 -28 -37 -47 -57 -63 -63 -54 -44 -34 -26 -21 -20 -22 -28 -37 -45 -45 -85];
      | B=[-50 -50 -50 -49 -45 -39 -33 -26 -21 -18 -17 -19 -22 -22 -26 -27 -25 -22 -16 -9 -3 2 6 6 4 1 1 -3 -4 -2 2 7 14 20 26 29 30 28 24 24 21 20 21 25 31 37 44 49 50 50 50 50];
      | C=[85 45 44 34 26 21 20 22 28 37 47 57 63 75 63 54 44 34 26 21 20 22 28 37 47 57 63 75 63 54 44 34 26 21 20 22 28 37 47 57 63 75 63 54 44 34 26 21 20 22 28 37 45 45 85];
      | D=[-50 -50 -50 -49 -45 -39 -33 -26 -21 -18 -17 -19 -22 -22 -22 -26 -27 -25 -22 -16 -9 -3 2 6 6 4 1 1 1 -3 -4 -2 2 7 14 20 26 29 30 28 24 24 24 21 20 21 25 31 37 44 49 50 50 50 50];
      | plot(-85,-100,85,100,A,B,C,D);
      | text(-50,-70, '1');text(40,-70, '2');
      | color('green')
      | port_label('Lconn',1,'+');port_label('Rconn',1,'+');
      | color('blue')
      | disp('N')
  L : PMIOPort  Tag=PMCPort  Side=Right
  S : PMIOPort  Port=2  Side=Left
  Isec : Outport
  Vsec : Outport  Port=2
  wires:
  tap/1 -> Tap Changing Transformer/1(Tap)
  Memory/1 -> Isec/1
  Memory1/1 -> Vsec/1
  " 1"/1 -> Memory/1
  CT/1 -> " 1"/1
  PT/1 -> "    "/1
  "    "/1 -> Memory1/1
  connections:
  Tap Changing Transformer/LConn2 -- Ground3/LConn1
  Tap Changing Transformer/LConn1 -- S/RConn1
  Tap Changing Transformer/RConn2 -- Ground2/LConn1
  CT/RConn1 -- L/RConn1
  PT/LConn1 -- CT/LConn1 -- Tap Changing Transformer/RConn1
  PT/LConn2 -- Ground1/LConn1

== system IEEE123bus_v2019b_Phasor_PI/Regulator 1/Single Phase SVR_A/Voltage Regulator Control ==
  Vm : Inport
  Constant : Constant  Value=RegulatorOn
  Tap Changer Control : Subsystem  mask(Tap Changer Control){MinMaxTap=TapMinMax, InitialPosition=InitialTap, MecDelay=TapSelectionTime}
      mask prompts: MinMaxTap "Minimum and maximum tap number [ Min  Max ] :"; InitialPosition "Initial tap position"; MecDelay "Mechanical delay time"
      mask init:
      | if MecDelay<=0,
      | 	MecDelay=1/60;
      | end
  Voltage regulator : Subsystem  mask{Vref=RegulatorVref*120, DeadBand=RegulatorDeadBand*120, TimeDelay=RegulatorDelay}
      mask prompts: Vref "Vref (on 120v base)"; DeadBand "Deadband (on 120v base)"; TimeDelay "Time delay (s)"
  Tap : Outport
  wires:
  Vm/1 -> Voltage regulator/1(Vmes (pu))
  Constant/1 -> Voltage regulator/3(RegOn)
  Tap Changer Control/2(Ready) -> Voltage regulator/2(Ready)
  Voltage regulator/1(Up) -> Tap Changer Control/1("Up ")
  Tap Changer Control/1(TapNo) -> Tap/1  "Tap"
  Voltage regulator/2(Down) -> Tap Changer Control/2("Down ")

== system IEEE123bus_v2019b_Phasor_PI/Regulator 1 Three Phase Ganged SVR/Single Phase SVR_A/Transformer with Taps ==
  note: Isec on CT Ratio base
  note: Vsec on Pt Ratio base
  tap : Inport
  "    " : Gain  Gain=(1/ptRatio)
  " 1" : Gain  Gain=(1/ctRatio)
  CT : powerlib/Measurements/Current Measurement  PhasorSimulation=on  OutputType=Complex  PSBequivalent=0
      settings: SourceProductName=Simscape Electrical
  Ground1 : powerlib/Elements/Ground  LConnTagsString=a
      settings: SourceProductName=Simscape Electrical
  Ground2 : powerlib/Elements/Ground  LConnTagsString=a
      settings: SourceProductName=Simscape Electrical
  Ground3 : powerlib/Elements/Ground  LConnTagsString=a
      settings: SourceProductName=Simscape Electrical
  Memory : Memory
  Memory1 : Memory
  PT : powerlib/Measurements/Voltage Measurement  PhasorSimulation=on  OutputType=Complex  PSBequivalent=0
      settings: SourceProductName=Simscape Electrical
  Tap Changing Transformer : Subsystem  mask(Tap Changing Transformer){}
      mask help: Implements a Tap changing two-winding ideal transformer with taps at secondary.
      mask Display:
      | A=[-85 -45 -44 -34 -26 -21 -20 -22 -28 -37 -47 -57 -63 -63 -54 -44 -34 -26 -21 -20 -22 -28 -37 -47 -57 -63 -63 -54 -44 -34 -26 -21 -20 -22 -28 -37 -47 -57 -63 -63 -54 -44 -34 -26 -21 -20 -22 -28 -37 -45 -45 -85];
      | B=[-50 -50 -50 -49 -45 -39 -33 -26 -21 -18 -17 -19 -22 -22 -26 -27 -25 -22 -16 -9 -3 2 6 6 4 1 1 -3 -4 -2 2 7 14 20 26 29 30 28 24 24 21 20 21 25 31 37 44 49 50 50 50 50];
      | C=[85 45 44 34 26 21 20 22 28 37 47 57 63 75 63 54 44 34 26 21 20 22 28 37 47 57 63 75 63 54 44 34 26 21 20 22 28 37 47 57 63 75 63 54 44 34 26 21 20 22 28 37 45 45 85];
      | D=[-50 -50 -50 -49 -45 -39 -33 -26 -21 -18 -17 -19 -22 -22 -22 -26 -27 -25 -22 -16 -9 -3 2 6 6 4 1 1 1 -3 -4 -2 2 7 14 20 26 29 30 28 24 24 24 21 20 21 25 31 37 44 49 50 50 50 50];
      | plot(-85,-100,85,100,A,B,C,D);
      | text(-50,-70, '1');text(40,-70, '2');
      | color('green')
      | port_label('Lconn',1,'+');port_label('Rconn',1,'+');
      | color('blue')
      | disp('N')
  L : PMIOPort  Tag=PMCPort  Side=Right
  S : PMIOPort  Port=2  Side=Left
  Isec : Outport
  Vsec : Outport  Port=2
  wires:
  tap/1 -> Tap Changing Transformer/1(Tap)
  Memory/1 -> Isec/1
  Memory1/1 -> Vsec/1
  " 1"/1 -> Memory/1
  CT/1 -> " 1"/1
  PT/1 -> "    "/1
  "    "/1 -> Memory1/1
  connections:
  Tap Changing Transformer/LConn2 -- Ground3/LConn1
  Tap Changing Transformer/LConn1 -- S/RConn1
  Tap Changing Transformer/RConn2 -- Ground2/LConn1
  CT/RConn1 -- L/RConn1
  PT/LConn1 -- CT/LConn1 -- Tap Changing Transformer/RConn1
  PT/LConn2 -- Ground1/LConn1

== system IEEE123bus_v2019b_Phasor_PI/Regulator 1 Three Phase Ganged SVR/Single Phase SVR_A/Voltage Regulator Control ==
  Vm : Inport
  Constant : Constant  Value=RegulatorOn
  Tap Changer Control : Subsystem  mask(Tap Changer Control){MinMaxTap=TapMinMax, InitialPosition=InitialTap, MecDelay=TapSelectionTime}
      mask prompts: MinMaxTap "Minimum and maximum tap number [ Min  Max ] :"; InitialPosition "Initial tap position"; MecDelay "Mechanical delay time"
      mask init:
      | if MecDelay<=0,
      | 	MecDelay=1/60;
      | end
  Voltage regulator : Subsystem  mask{Vref=RegulatorVref*120, DeadBand=RegulatorDeadBand*120, TimeDelay=RegulatorDelay}
      mask prompts: Vref "Vref (on 120v base)"; DeadBand "Deadband (on 120v base)"; TimeDelay "Time delay (s)"
  Tap : Outport
  wires:
  Vm/1 -> Voltage regulator/1(Vmes (pu))
  Constant/1 -> Voltage regulator/3(RegOn)
  Tap Changer Control/2(Ready) -> Voltage regulator/2(Ready)
  Voltage regulator/1(Up) -> Tap Changer Control/1("Up ")
  Tap Changer Control/1(TapNo) -> Tap/1  "Tap"
  Voltage regulator/2(Down) -> Tap Changer Control/2("Down ")

== system IEEE123bus_v2019b_Phasor_PI/Regulator 1 Three Phase Ganged SVR/Single Phase SVR_B/Transformer with Taps ==
  note: Isec on CT Ratio base
  note: Vsec on Pt Ratio base
  tap : Inport
  "    " : Gain  Gain=(1/ptRatio)
  " 1" : Gain  Gain=(1/ctRatio)
  CT : powerlib/Measurements/Current Measurement  PhasorSimulation=on  OutputType=Complex  PSBequivalent=0
      settings: SourceProductName=Simscape Electrical
  Ground1 : powerlib/Elements/Ground  LConnTagsString=a
      settings: SourceProductName=Simscape Electrical
  Ground2 : powerlib/Elements/Ground  LConnTagsString=a
      settings: SourceProductName=Simscape Electrical
  Ground3 : powerlib/Elements/Ground  LConnTagsString=a
      settings: SourceProductName=Simscape Electrical
  Memory : Memory
  Memory1 : Memory
  PT : powerlib/Measurements/Voltage Measurement  PhasorSimulation=on  OutputType=Complex  PSBequivalent=0
      settings: SourceProductName=Simscape Electrical
  Tap Changing Transformer : Subsystem  mask(Tap Changing Transformer){}
      mask help: Implements a Tap changing two-winding ideal transformer with taps at secondary.
      mask Display:
      | A=[-85 -45 -44 -34 -26 -21 -20 -22 -28 -37 -47 -57 -63 -63 -54 -44 -34 -26 -21 -20 -22 -28 -37 -47 -57 -63 -63 -54 -44 -34 -26 -21 -20 -22 -28 -37 -47 -57 -63 -63 -54 -44 -34 -26 -21 -20 -22 -28 -37 -45 -45 -85];
      | B=[-50 -50 -50 -49 -45 -39 -33 -26 -21 -18 -17 -19 -22 -22 -26 -27 -25 -22 -16 -9 -3 2 6 6 4 1 1 -3 -4 -2 2 7 14 20 26 29 30 28 24 24 21 20 21 25 31 37 44 49 50 50 50 50];
      | C=[85 45 44 34 26 21 20 22 28 37 47 57 63 75 63 54 44 34 26 21 20 22 28 37 47 57 63 75 63 54 44 34 26 21 20 22 28 37 47 57 63 75 63 54 44 34 26 21 20 22 28 37 45 45 85];
      | D=[-50 -50 -50 -49 -45 -39 -33 -26 -21 -18 -17 -19 -22 -22 -22 -26 -27 -25 -22 -16 -9 -3 2 6 6 4 1 1 1 -3 -4 -2 2 7 14 20 26 29 30 28 24 24 24 21 20 21 25 31 37 44 49 50 50 50 50];
      | plot(-85,-100,85,100,A,B,C,D);
      | text(-50,-70, '1');text(40,-70, '2');
      | color('green')
      | port_label('Lconn',1,'+');port_label('Rconn',1,'+');
      | color('blue')
      | disp('N')
  L : PMIOPort  Tag=PMCPort  Side=Right
  S : PMIOPort  Port=2  Side=Left
  Isec : Outport
  Vsec : Outport  Port=2
  wires:
  tap/1 -> Tap Changing Transformer/1(Tap)
  Memory/1 -> Isec/1
  Memory1/1 -> Vsec/1
  " 1"/1 -> Memory/1
  CT/1 -> " 1"/1
  PT/1 -> "    "/1
  "    "/1 -> Memory1/1
  connections:
  Tap Changing Transformer/LConn2 -- Ground3/LConn1
  Tap Changing Transformer/LConn1 -- S/RConn1
  Tap Changing Transformer/RConn2 -- Ground2/LConn1
  CT/RConn1 -- L/RConn1
  PT/LConn1 -- CT/LConn1 -- Tap Changing Transformer/RConn1
  PT/LConn2 -- Ground1/LConn1

== system IEEE123bus_v2019b_Phasor_PI/Regulator 1 Three Phase Ganged SVR/Single Phase SVR_B/Voltage Regulator Control ==
  Vm : Inport
  Constant : Constant  Value=RegulatorOn
  Tap Changer Control : Subsystem  mask(Tap Changer Control){MinMaxTap=TapMinMax, InitialPosition=InitialTap, MecDelay=TapSelectionTime}
      mask prompts: MinMaxTap "Minimum and maximum tap number [ Min  Max ] :"; InitialPosition "Initial tap position"; MecDelay "Mechanical delay time"
      mask init:
      | if MecDelay<=0,
      | 	MecDelay=1/60;
      | end
  Voltage regulator : Subsystem  mask{Vref=RegulatorVref*120, DeadBand=RegulatorDeadBand*120, TimeDelay=RegulatorDelay}
      mask prompts: Vref "Vref (on 120v base)"; DeadBand "Deadband (on 120v base)"; TimeDelay "Time delay (s)"
  Tap : Outport
  wires:
  Vm/1 -> Voltage regulator/1(Vmes (pu))
  Constant/1 -> Voltage regulator/3(RegOn)
  Tap Changer Control/2(Ready) -> Voltage regulator/2(Ready)
  Voltage regulator/1(Up) -> Tap Changer Control/1("Up ")
  Tap Changer Control/1(TapNo) -> Tap/1  "Tap"
  Voltage regulator/2(Down) -> Tap Changer Control/2("Down ")

== system IEEE123bus_v2019b_Phasor_PI/Regulator 1 Three Phase Ganged SVR/Single Phase SVR_C/Transformer with Taps ==
  note: Isec on CT Ratio base
  note: Vsec on Pt Ratio base
  tap : Inport
  "    " : Gain  Gain=(1/ptRatio)
  " 1" : Gain  Gain=(1/ctRatio)
  CT : powerlib/Measurements/Current Measurement  PhasorSimulation=on  OutputType=Complex  PSBequivalent=0
      settings: SourceProductName=Simscape Electrical
  Ground1 : powerlib/Elements/Ground  LConnTagsString=a
      settings: SourceProductName=Simscape Electrical
  Ground2 : powerlib/Elements/Ground  LConnTagsString=a
      settings: SourceProductName=Simscape Electrical
  Ground3 : powerlib/Elements/Ground  LConnTagsString=a
      settings: SourceProductName=Simscape Electrical
  Memory : Memory
  Memory1 : Memory
  PT : powerlib/Measurements/Voltage Measurement  PhasorSimulation=on  OutputType=Complex  PSBequivalent=0
      settings: SourceProductName=Simscape Electrical
  Tap Changing Transformer : Subsystem  mask(Tap Changing Transformer){}
      mask help: Implements a Tap changing two-winding ideal transformer with taps at secondary.
      mask Display:
      | A=[-85 -45 -44 -34 -26 -21 -20 -22 -28 -37 -47 -57 -63 -63 -54 -44 -34 -26 -21 -20 -22 -28 -37 -47 -57 -63 -63 -54 -44 -34 -26 -21 -20 -22 -28 -37 -47 -57 -63 -63 -54 -44 -34 -26 -21 -20 -22 -28 -37 -45 -45 -85];
      | B=[-50 -50 -50 -49 -45 -39 -33 -26 -21 -18 -17 -19 -22 -22 -26 -27 -25 -22 -16 -9 -3 2 6 6 4 1 1 -3 -4 -2 2 7 14 20 26 29 30 28 24 24 21 20 21 25 31 37 44 49 50 50 50 50];
      | C=[85 45 44 34 26 21 20 22 28 37 47 57 63 75 63 54 44 34 26 21 20 22 28 37 47 57 63 75 63 54 44 34 26 21 20 22 28 37 47 57 63 75 63 54 44 34 26 21 20 22 28 37 45 45 85];
      | D=[-50 -50 -50 -49 -45 -39 -33 -26 -21 -18 -17 -19 -22 -22 -22 -26 -27 -25 -22 -16 -9 -3 2 6 6 4 1 1 1 -3 -4 -2 2 7 14 20 26 29 30 28 24 24 24 21 20 21 25 31 37 44 49 50 50 50 50];
      | plot(-85,-100,85,100,A,B,C,D);
      | text(-50,-70, '1');text(40,-70, '2');
      | color('green')
      | port_label('Lconn',1,'+');port_label('Rconn',1,'+');
      | color('blue')
      | disp('N')
  L : PMIOPort  Tag=PMCPort  Side=Right
  S : PMIOPort  Port=2  Side=Left
  Isec : Outport
  Vsec : Outport  Port=2
  wires:
  tap/1 -> Tap Changing Transformer/1(Tap)
  Memory/1 -> Isec/1
  Memory1/1 -> Vsec/1
  " 1"/1 -> Memory/1
  CT/1 -> " 1"/1
  PT/1 -> "    "/1
  "    "/1 -> Memory1/1
  connections:
  Tap Changing Transformer/LConn2 -- Ground3/LConn1
  Tap Changing Transformer/LConn1 -- S/RConn1
  Tap Changing Transformer/RConn2 -- Ground2/LConn1
  CT/RConn1 -- L/RConn1
  PT/LConn1 -- CT/LConn1 -- Tap Changing Transformer/RConn1
  PT/LConn2 -- Ground1/LConn1

== system IEEE123bus_v2019b_Phasor_PI/Regulator 1 Three Phase Ganged SVR/Single Phase SVR_C/Voltage Regulator Control ==
  Vm : Inport
  Constant : Constant  Value=RegulatorOn
  Tap Changer Control : Subsystem  mask(Tap Changer Control){MinMaxTap=TapMinMax, InitialPosition=InitialTap, MecDelay=TapSelectionTime}
      mask prompts: MinMaxTap "Minimum and maximum tap number [ Min  Max ] :"; InitialPosition "Initial tap position"; MecDelay "Mechanical delay time"
      mask init:
      | if MecDelay<=0,
      | 	MecDelay=1/60;
      | end
  Voltage regulator : Subsystem  mask{Vref=RegulatorVref*120, DeadBand=RegulatorDeadBand*120, TimeDelay=RegulatorDelay}
      mask prompts: Vref "Vref (on 120v base)"; DeadBand "Deadband (on 120v base)"; TimeDelay "Time delay (s)"
  Tap : Outport
  wires:
  Vm/1 -> Voltage regulator/1(Vmes (pu))
  Constant/1 -> Voltage regulator/3(RegOn)
  Tap Changer Control/2(Ready) -> Voltage regulator/2(Ready)
  Voltage regulator/1(Up) -> Tap Changer Control/1("Up ")
  Tap Changer Control/1(TapNo) -> Tap/1  "Tap"
  Voltage regulator/2(Down) -> Tap Changer Control/2("Down ")

== system IEEE123bus_v2019b_Phasor_PI/Regulator 3/Single Phase SVR_A/Line Drop Compensator ==
  note: Vm=Vsec-Isec(Rc+jXc)
  Isec : Inport
  Vsec : Inport  Port=2
  Abs1 : Abs
  Complex to Magnitude-Angle1 : ComplexToMagnitudeAngle
  Complex to Magnitude-Angle2 : ComplexToMagnitudeAngle
  Display{,1..3} (4 alike) : Display
  Gain1 : Gain  Gain=ptRatio
  Gain2 : Gain  Gain=1/120
  Gain3 : Gain  Gain=1/(4160/sqrt(3))
  Gain4 : Gain  Gain=1/sqrt(2)
  Gain5 : Gain  Gain=Rc+j*Xc
  Gain6 : Gain  Gain=1/sqrt(2)
  Gain7 : Gain  Gain=ctRatio
  Sum1 : Sum  Inputs=|+-
  Vm : Outport
  wires:
  Gain5/1 -> Sum1/2
  Gain6/1 -> Complex to Magnitude-Angle1/1, Sum1/1
  Vsec/1 -> Gain6/1
  Isec/1 -> Gain4/1
  Sum1/1 -> Abs1/1
  Abs1/1 -> Gain2/1, Display/1, Vm/1
  Complex to Magnitude-Angle1/1 -> Gain1/1
  Gain1/1 -> Gain3/1
  Gain2/1 -> Display2/1
  Gain3/1 -> Display1/1
  Gain4/1 -> Complex to Magnitude-Angle2/1, Gain5/1
  Gain7/1 -> Display3/1
  Complex to Magnitude-Angle2/1 -> Gain7/1

== system IEEE123bus_v2019b_Phasor_PI/Regulator 3/Single Phase SVR_A/Transformer with Taps ==
  note: Isec on CT Ratio base
  note: Vsec on Pt Ratio base
  tap : Inport
  "    " : Gain  Gain=(1/ptRatio)
  " 1" : Gain  Gain=(1/ctRatio)
  CT : powerlib/Measurements/Current Measurement  PhasorSimulation=on  OutputType=Complex  PSBequivalent=0
      settings: SourceProductName=Simscape Electrical
  Ground1 : powerlib/Elements/Ground  LConnTagsString=a
      settings: SourceProductName=Simscape Electrical
  Ground2 : powerlib/Elements/Ground  LConnTagsString=a
      settings: SourceProductName=Simscape Electrical
  Ground3 : powerlib/Elements/Ground  LConnTagsString=a
      settings: SourceProductName=Simscape Electrical
  Memory : Memory
  Memory1 : Memory
  PT : powerlib/Measurements/Voltage Measurement  PhasorSimulation=on  OutputType=Complex  PSBequivalent=0
      settings: SourceProductName=Simscape Electrical
  Tap Changing Transformer : Subsystem  mask(Tap Changing Transformer){}
      mask help: Implements a Tap changing two-winding ideal transformer with taps at secondary.
      mask Display:
      | A=[-85 -45 -44 -34 -26 -21 -20 -22 -28 -37 -47 -57 -63 -63 -54 -44 -34 -26 -21 -20 -22 -28 -37 -47 -57 -63 -63 -54 -44 -34 -26 -21 -20 -22 -28 -37 -47 -57 -63 -63 -54 -44 -34 -26 -21 -20 -22 -28 -37 -45 -45 -85];
      | B=[-50 -50 -50 -49 -45 -39 -33 -26 -21 -18 -17 -19 -22 -22 -26 -27 -25 -22 -16 -9 -3 2 6 6 4 1 1 -3 -4 -2 2 7 14 20 26 29 30 28 24 24 21 20 21 25 31 37 44 49 50 50 50 50];
      | C=[85 45 44 34 26 21 20 22 28 37 47 57 63 75 63 54 44 34 26 21 20 22 28 37 47 57 63 75 63 54 44 34 26 21 20 22 28 37 47 57 63 75 63 54 44 34 26 21 20 22 28 37 45 45 85];
      | D=[-50 -50 -50 -49 -45 -39 -33 -26 -21 -18 -17 -19 -22 -22 -22 -26 -27 -25 -22 -16 -9 -3 2 6 6 4 1 1 1 -3 -4 -2 2 7 14 20 26 29 30 28 24 24 24 21 20 21 25 31 37 44 49 50 50 50 50];
      | plot(-85,-100,85,100,A,B,C,D);
      | text(-50,-70, '1');text(40,-70, '2');
      | color('green')
      | port_label('Lconn',1,'+');port_label('Rconn',1,'+');
      | color('blue')
      | disp('N')
  L : PMIOPort  Tag=PMCPort  Side=Right
  S : PMIOPort  Port=2  Side=Left
  Isec : Outport
  Vsec : Outport  Port=2
  wires:
  tap/1 -> Tap Changing Transformer/1(Tap)
  Memory/1 -> Isec/1
  Memory1/1 -> Vsec/1
  " 1"/1 -> Memory/1
  CT/1 -> " 1"/1
  PT/1 -> "    "/1
  "    "/1 -> Memory1/1
  connections:
  Tap Changing Transformer/LConn2 -- Ground3/LConn1
  Tap Changing Transformer/LConn1 -- S/RConn1
  Tap Changing Transformer/RConn2 -- Ground2/LConn1
  CT/RConn1 -- L/RConn1
  PT/LConn1 -- CT/LConn1 -- Tap Changing Transformer/RConn1
  PT/LConn2 -- Ground1/LConn1

== system IEEE123bus_v2019b_Phasor_PI/Regulator 3/Single Phase SVR_A/Voltage Regulator Control ==
  Vm : Inport
  Constant : Constant  Value=RegulatorOn
  Tap Changer Control : Subsystem  mask(Tap Changer Control){MinMaxTap=TapMinMax, InitialPosition=InitialTap, MecDelay=TapSelectionTime}
      mask prompts: MinMaxTap "Minimum and maximum tap number [ Min  Max ] :"; InitialPosition "Initial tap position"; MecDelay "Mechanical delay time"
      mask init:
      | if MecDelay<=0,
      | 	MecDelay=1/60;
      | end
  Voltage regulator : Subsystem  mask{Vref=RegulatorVref*120, DeadBand=RegulatorDeadBand*120, TimeDelay=RegulatorDelay}
      mask prompts: Vref "Vref (on 120v base)"; DeadBand "Deadband (on 120v base)"; TimeDelay "Time delay (s)"
  Tap : Outport
  wires:
  Vm/1 -> Voltage regulator/1(Vmes (pu))
  Constant/1 -> Voltage regulator/3(RegOn)
  Tap Changer Control/2(Ready) -> Voltage regulator/2(Ready)
  Voltage regulator/1(Up) -> Tap Changer Control/1("Up ")
  Tap Changer Control/1(TapNo) -> Tap/1  "Tap"
  Voltage regulator/2(Down) -> Tap Changer Control/2("Down ")

== system IEEE123bus_v2019b_Phasor_PI/Regulator 3/Single Phase SVR_C/Line Drop Compensator ==
  note: Vm=Vsec-Isec(Rc+jXc)
  Isec : Inport
  Vsec : Inport  Port=2
  Abs1 : Abs
  Complex to Magnitude-Angle1 : ComplexToMagnitudeAngle
  Complex to Magnitude-Angle2 : ComplexToMagnitudeAngle
  Display{,1..3} (4 alike) : Display
  Gain1 : Gain  Gain=ptRatio
  Gain2 : Gain  Gain=1/120
  Gain3 : Gain  Gain=1/(4160/sqrt(3))
  Gain4 : Gain  Gain=1/sqrt(2)
  Gain5 : Gain  Gain=Rc+j*Xc
  Gain6 : Gain  Gain=1/sqrt(2)
  Gain7 : Gain  Gain=ctRatio
  Sum1 : Sum  Inputs=|+-
  Vm : Outport
  wires:
  Gain5/1 -> Sum1/2
  Vsec/1 -> Gain6/1
  Isec/1 -> Gain4/1
  Sum1/1 -> Abs1/1
  Gain6/1 -> Complex to Magnitude-Angle1/1, Sum1/1
  Gain3/1 -> Display1/1
  Gain2/1 -> Display2/1
  Gain1/1 -> Gain3/1
  Complex to Magnitude-Angle1/1 -> Gain1/1
  Abs1/1 -> Gain2/1, Display/1, Vm/1
  Complex to Magnitude-Angle2/1 -> Gain7/1
  Gain7/1 -> Display3/1
  Gain4/1 -> Complex to Magnitude-Angle2/1, Gain5/1

== system IEEE123bus_v2019b_Phasor_PI/Regulator 3/Single Phase SVR_C/Transformer with Taps ==
  note: Isec on CT Ratio base
  note: Vsec on Pt Ratio base
  tap : Inport
  "    " : Gain  Gain=(1/ptRatio)
  " 1" : Gain  Gain=(1/ctRatio)
  CT : powerlib/Measurements/Current Measurement  PhasorSimulation=on  OutputType=Complex  PSBequivalent=0
      settings: SourceProductName=Simscape Electrical
  Ground1 : powerlib/Elements/Ground  LConnTagsString=a
      settings: SourceProductName=Simscape Electrical
  Ground2 : powerlib/Elements/Ground  LConnTagsString=a
      settings: SourceProductName=Simscape Electrical
  Ground3 : powerlib/Elements/Ground  LConnTagsString=a
      settings: SourceProductName=Simscape Electrical
  Memory : Memory
  Memory1 : Memory
  PT : powerlib/Measurements/Voltage Measurement  PhasorSimulation=on  OutputType=Complex  PSBequivalent=0
      settings: SourceProductName=Simscape Electrical
  Tap Changing Transformer : Subsystem  mask(Tap Changing Transformer){}
      mask help: Implements a Tap changing two-winding ideal transformer with taps at secondary.
      mask Display:
      | A=[-85 -45 -44 -34 -26 -21 -20 -22 -28 -37 -47 -57 -63 -63 -54 -44 -34 -26 -21 -20 -22 -28 -37 -47 -57 -63 -63 -54 -44 -34 -26 -21 -20 -22 -28 -37 -47 -57 -63 -63 -54 -44 -34 -26 -21 -20 -22 -28 -37 -45 -45 -85];
      | B=[-50 -50 -50 -49 -45 -39 -33 -26 -21 -18 -17 -19 -22 -22 -26 -27 -25 -22 -16 -9 -3 2 6 6 4 1 1 -3 -4 -2 2 7 14 20 26 29 30 28 24 24 21 20 21 25 31 37 44 49 50 50 50 50];
      | C=[85 45 44 34 26 21 20 22 28 37 47 57 63 75 63 54 44 34 26 21 20 22 28 37 47 57 63 75 63 54 44 34 26 21 20 22 28 37 47 57 63 75 63 54 44 34 26 21 20 22 28 37 45 45 85];
      | D=[-50 -50 -50 -49 -45 -39 -33 -26 -21 -18 -17 -19 -22 -22 -22 -26 -27 -25 -22 -16 -9 -3 2 6 6 4 1 1 1 -3 -4 -2 2 7 14 20 26 29 30 28 24 24 24 21 20 21 25 31 37 44 49 50 50 50 50];
      | plot(-85,-100,85,100,A,B,C,D);
      | text(-50,-70, '1');text(40,-70, '2');
      | color('green')
      | port_label('Lconn',1,'+');port_label('Rconn',1,'+');
      | color('blue')
      | disp('N')
  L : PMIOPort  Tag=PMCPort  Side=Right
  S : PMIOPort  Port=2  Side=Left
  Isec : Outport
  Vsec : Outport  Port=2
  wires:
  tap/1 -> Tap Changing Transformer/1(Tap)
  Memory/1 -> Isec/1
  Memory1/1 -> Vsec/1
  " 1"/1 -> Memory/1
  CT/1 -> " 1"/1
  PT/1 -> "    "/1
  "    "/1 -> Memory1/1
  connections:
  Tap Changing Transformer/LConn2 -- Ground3/LConn1
  Tap Changing Transformer/LConn1 -- S/RConn1
  Tap Changing Transformer/RConn2 -- Ground2/LConn1
  CT/RConn1 -- L/RConn1
  PT/LConn1 -- CT/LConn1 -- Tap Changing Transformer/RConn1
  PT/LConn2 -- Ground1/LConn1
